simulink model "Buck_VMC"  (R2024a)
settings: Solver=VariableStepAuto  StartTime=0.0  StopTime=.024  RelTol=1e-3
values from neighbouring files (symbols this model uses):
  C = 500*10^(-6)    (= 0.0005)    [parameters.m]
  Fp_PD = Fc*sqrt((1+sind(reqPM))/(1-sind(reqPM)))    [parameters.m]
  Fz_PD = Fc*sqrt((1-sind(reqPM))/(1+sind(reqPM)))    [parameters.m]
  Gco_PD = sqrt(Fz_PD/Fp_PD)/reqGain    [parameters.m]
  L = 50*10^(-6)    (= 5e-05)    [parameters.m]
  R = 3    [parameters.m]
  R1 = 20*10^(3)    (= 20000)    [parameters.m]
  R2 = 10*10^(3)    (= 10000)    [parameters.m]
  Vin = 28    [parameters.m]
  WL = (Fc/10)*2*pi    (= 3141.59265359)    [parameters.m]
libraries: spsSeriesRLCBranchLib x5, spsVoltageMeasurementLib x2, spsDCVoltageSourceLib x1, spsDiodeLib x1, spsMosfetLib x1, simulink x1, sps_lib x1
settings Model: Creator=User  LastModifiedBy=User

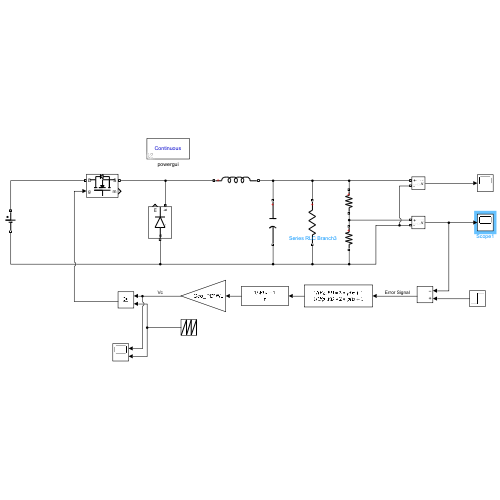
[thumbnail: Simulink's stored preview of the top-level diagram]
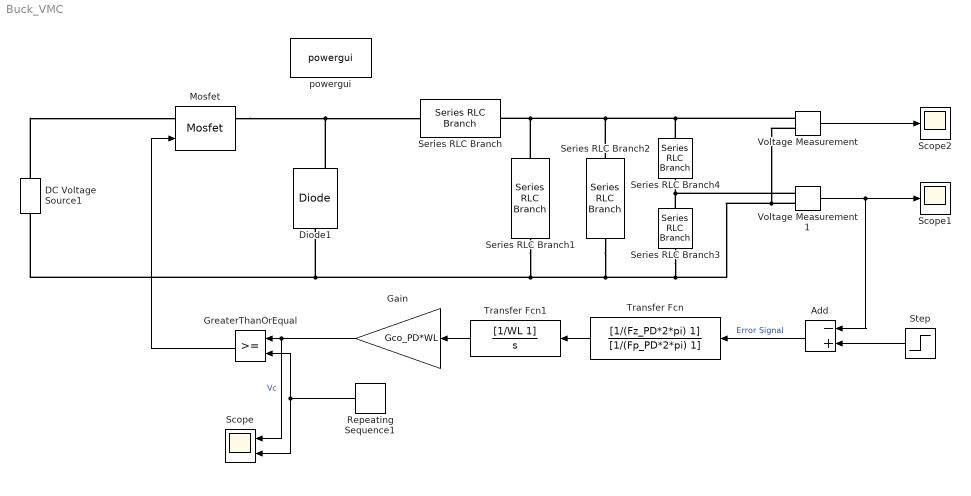
== system Buck_VMC ==
  Add : Sum  Inputs=-+
  DC Voltage Source1 : spsDCVoltageSourceLib/DC Voltage Source  Amplitude=Vin  Measurements=None
  Diode1 : spsDiodeLib/Diode  Ron=0.001  Lon=0  Vf=0.8  IC=0  UseSnubber=0  Rs=500  Cs=250e-9  Measurements=on
  Gain : Gain  Gain=Gco_PD*WL
  GreaterThanOrEqual : RelationalOperator  OutDataTypeStr=boolean  RndMeth=Simplest  InputSameDT=off
  Mosfet : spsMosfetLib/Mosfet  Ron=0.1  Lon=0  Rd=0.01  Vfd=0  IC=0  Rs=1e5  Cs=inf  Measurements=on
  Repeating Sequence1 : simulink/Sources/Repeating Sequence  rep_seq_t=[0 1]/100000  rep_seq_y=[0 1]
  Scope : Scope  NumInputPorts=2
  Scope1 : Scope
  Scope2 : Scope
  Series RLC Branch : spsSeriesRLCBranchLib/Series RLC Branch  LConnTagsString=__new0  RConnTagsString=__new0  BranchType=L  Resistance=1  Inductance=L  SetiL0=off  InitialCurrent=0  Capacitance=1e-6  Setx0=off  InitialVoltage=0  Measurements=None
  Series RLC Branch1 : spsSeriesRLCBranchLib/Series RLC Branch  LConnTagsString=__new0  RConnTagsString=__new0  BranchType=C  Resistance=1  Inductance=L  SetiL0=off  InitialCurrent=0  Capacitance=C  Setx0=off  InitialVoltage=0  Measurements=None
  Series RLC Branch2 : spsSeriesRLCBranchLib/Series RLC Branch  LConnTagsString=__new0  RConnTagsString=__new0  BranchType=R  Resistance=R  Inductance=L  SetiL0=off  InitialCurrent=0  Capacitance=C  Setx0=off  InitialVoltage=0  Measurements=None
  Series RLC Branch3 : spsSeriesRLCBranchLib/Series RLC Branch  LConnTagsString=__new0  RConnTagsString=__new0  BranchType=R  Resistance=R2  Inductance=L  SetiL0=off  InitialCurrent=0  Capacitance=C  Setx0=off  InitialVoltage=0  Measurements=None
  Series RLC Branch4 : spsSeriesRLCBranchLib/Series RLC Branch  LConnTagsString=__new0  RConnTagsString=__new0  BranchType=R  Resistance=R1  Inductance=L  SetiL0=off  InitialCurrent=0  Capacitance=C  Setx0=off  InitialVoltage=0  Measurements=None
  Step : Step  Time=.012  Before=4  After=5  SampleTime=0
  Transfer Fcn : TransferFcn  Numerator=[1/(Fz_PD*2*pi) 1]  Denominator=[1/(Fp_PD*2*pi) 1]
  Transfer Fcn1 : TransferFcn  Numerator=[1/WL 1]  Denominator=[1 0]
  Voltage Measurement : spsVoltageMeasurementLib/Voltage Measurement  PhasorSimulation=off  OutputType=Complex  PSBequivalent=0
  Voltage Measurement1 : spsVoltageMeasurementLib/Voltage Measurement  PhasorSimulation=off  OutputType=Complex  PSBequivalent=0
  powergui : sps_lib/powergui  Priority=1  SimulationMode=Continuous  SampleTime=50e-6  frequency=60  Iterations=50  frequencyindice=0  Pbase=100e6  ErrMax=1e-4  UnitsV=kV  UnitsW=MW  buscounter=0  FunctionMessages=off  echomessages=off  EnableUseOfTLC=off  CurrentSourceSwitches=off  DisableSnubberDevices=on  DisableRonSwitches=on  DisableVfSwitches=on  DisplayEquations=off  AutomaticDiscreteSolvers=off  SolverType=Tustin/Backward Euler (TBE)  Interpol=off  ExternalGateDelay=off  methode=off  Ts=100  x0status=blocks  SPID=on  SwTol=0  HookPort=off  NonlinearTolerance=1e-4  nMaxIteration=100  ContinueOnMaxIteration=off  RestoreLinks=warning  ResistiveCurrentMeasurement=off  Frange=[0:2:500]  Ylog=off  Xlog=on  ShowGrid=off  save=off  variable=ZData  structure=0  ZoomFFT=off  StartTime=0.0  cycles=1  DisplayStyle=1  fundamental=60  FreqAxis=off  MaxFrequency=1000  frequencyindicesteady=1  RmsSteady=1  display=off
  wires:
  Add/1 -> Transfer Fcn/1  "Error Signal"
  Transfer Fcn1/1 -> Gain/1
  Gain/1 -> Scope/1, GreaterThanOrEqual/1  "Vc"
  GreaterThanOrEqual/1 -> Mosfet/1
  Transfer Fcn/1 -> Transfer Fcn1/1
  Voltage Measurement1/1 -> Scope1/1, Add/1
  Repeating Sequence1/1 -> Scope/2, GreaterThanOrEqual/2
  Voltage Measurement/1 -> Scope2/1
  Step/1 -> Add/2
  connections:
  Mosfet/RConn1 -- Series RLC Branch/LConn1 -- Diode1/RConn1
  DC Voltage Source1/RConn1 -- Mosfet/LConn1
  Series RLC Branch1/LConn1 -- Series RLC Branch4/LConn1 -- Voltage Measurement/LConn1 -- Series RLC Branch2/LConn1 -- Series RLC Branch/RConn1
  Series RLC Branch1/RConn1 -- Voltage Measurement/LConn2 -- Voltage Measurement1/LConn2 -- Series RLC Branch3/RConn1 -- Series RLC Branch2/RConn1 -- DC Voltage Source1/LConn1 -- Diode1/LConn1
  Series RLC Branch3/LConn1 -- Voltage Measurement1/LConn1 -- Series RLC Branch4/RConn1
